simulink model "q5_a_simulink_PD"  (R2013a)
settings: Solver=ode45  StartTime=0.0  StopTime=2  RelTol=1e-3
settings Model: Creator=obrien94  LastModifiedBy=obrien94
settings DebuggingCC: SolverPrmCheckMsg=none

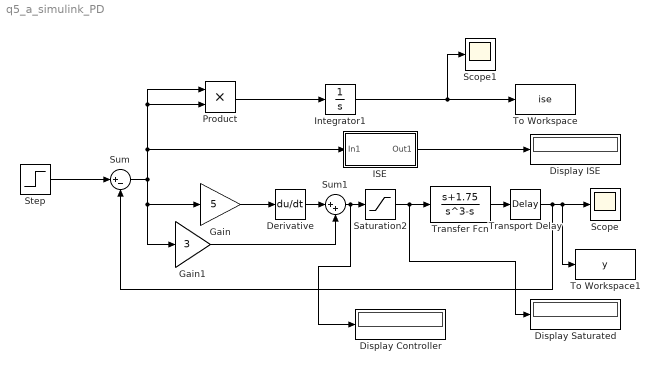
== system q5_a_simulink_PD ==
  Derivative : Derivative
  Display Controller : Display
  Display ISE : Display
  Display Saturated : Display
  Gain : Gain  Gain=5
  Gain1 : Gain  Gain=3
  ISE : Subsystem
      mask help:
      | ISE performance index
      |
      | output = int (input)^2 dt
      mask Display:
      | disp('ISE')
      | port_label('input',1,'e')
      | port_label('output',1,'ise')
  Integrator1 : Integrator
  Product : Product
  Saturation2 : Saturate  UpperLimit=5  LowerLimit=5
  Scope : Scope
  Scope1 : Scope
  Step : Step  SampleTime=0
  Sum : Sum  Inputs=|+-
  Sum1 : Sum  Inputs=|++
  To Workspace : ToWorkspace  VariableName=ise  SampleTime=-1
  To Workspace1 : ToWorkspace  VariableName=y  SampleTime=-1  SaveFormat=Timeseries
  Transfer Fcn : TransferFcn  Numerator=[1 1.75]  Denominator=[1 0 -1 0]
  Transport Delay : TransportDelay  DelayTime=0.00001
  wires:
  Step/1 -> Sum/1
  Sum/1 -> Gain1/1, Gain/1, Product/1, Product/2, ISE/1(In1)
  Product/1 -> Integrator1/1
  Integrator1/1 -> Scope1/1, To Workspace/1
  Derivative/1 -> Sum1/1
  ISE/1(Out1) -> Display ISE/1
  Sum1/1 -> Display Controller/1, Saturation2/1
  Gain/1 -> Derivative/1
  Gain1/1 -> Sum1/2
  Transfer Fcn/1 -> Transport Delay/1
  Saturation2/1 -> Display Saturated/1, Transfer Fcn/1
  Transport Delay/1 -> To Workspace1/1, Scope/1, Sum/2

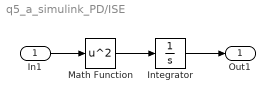
== system q5_a_simulink_PD/ISE ==
  In1 : Inport
  Integrator : Integrator
  Math Function : Math  Operator=square  SaturateOnIntegerOverflow=on
  Out1 : Outport
  wires:
  Math Function/1 -> Integrator/1
  Integrator/1 -> Out1/1
  In1/1 -> Math Function/1
